simulink model "car_model"  (R2022b)
settings: Solver=VariableStepAuto  StartTime=0.0  StopTime=30  RelTol=1e-3
values from neighbouring files (symbols this model uses):
  X = Chassis_Signals.InertFrm.Cg.Disp.X.Data(:)    [Simulation_Data_Parse.m]    (also in Vehicle_Sim_Parse.m)
  Y = Chassis_Signals.InertFrm.Cg.Disp.Y.Data(:)    [Simulation_Data_Parse.m]    (also in Vehicle_Sim_Parse.m)
undefined symbols (not defined in the file or in its folder): ABS_MAX_TORQUE, ABS_MAX_TRQ_CMD, ABS_MIN_TORQUE, acc_IC, ACCELERATION_MAX, ActSuspDutyCycle, Aeq_left, Aeq_right, alpha_error, ang_acc_hystersesis, ang_IC, ang_vel_IC, area_air, axb, battery_current_IC, BATTERY_CURRENT_MAX, BATTERY_CURRENT_MIN, battery_FT_IC, battery_T_IC, BATTERY_TEMPERATURE_MAX, BATTERY_TEMPERATURE_MIN, battery_voltage_IC, BATTERY_VOLTAGE_MAX, BATTERY_VOLTAGE_MIN, Brake_Pressure_IC, ccl_IC, CENTER_STEER_ANGLE_MAX, covA, covarience_matrix_IC, covG, covM, covP, covV, cy_sweep, dB, dcl_IC, DCL_MAX, DCL_MIN, deadband_angle, dIndex, DiscIntNeverNeededParam, disk_abore, driver_t, dt_OFF, dt_ON, dTx, dx, dZ, F0z, forward_look_straight, forward_look_turn, fusion_t, fusion_t_sim, Fz_IC, Fz_sweep, g, gearbox_efficiency, gps_counter_IC, gps_ratio, gr ... (+105)
libraries: fl_lib x62, nesl_utility x16, vehdynlibtire x10, vehdynlibsuspension x8, simulink x5, autolibutils x5, sharedtransform x5, EngineCoolingComponents_lib x4, slpidlib x3, SimscapeFluids_lib x3, dspstat3 x2, shared6dof x2
(part 10 of 10)

== system car_model/Vehicle Model/Wheels and Tires/VDBS/Tires/MF Tires Vector ==
  DriveTorque : Inport
  Brake Pedal : Inport  Port=2
  r : Inport  Port=3
  Vx : Inport  Port=4
  Vy : Inport  Port=5
  Camber : Inport  Port=6
  Press : Inport  Port=7  Unit=Pa
  lambda : Inport  Port=8  Unit=1
  Gnd : Inport  Port=9
  FzSusp : Inport  Port=10
  Combined Slip Wheel 2DOF : vehdynlibtire/Combined Slip Wheel 2DOF  plySteer=on  turnslip=on  tireType=External file  BrakeType=Disc  mu_static=mu_static  mu_kinetic=mu_kinetic  disk_abore=disk_abore  Rm=Rm  num_pads=num_pads  drum_abore=0.0508  drum_a=0.123  drum_c=0.212  drum_r=0.15  drum_theta1=0  drum_theta2=126  brake_p_bpt=[1 11.4736842105263 21.9473684210526 32.4210526315789 42.8947368421053 53.3684210526316 63.8421052631579 74.3157894736842 84.7894736842105 95.2631578947368 105.736842105263 116.210526315789 126.684210526316 137.157894736842 147.631578947368 158.105263157895 168.578947368421 179.052631578947 189.526315789474 200]  brake_n_bpt=[0 52.6315789473684 105.263157894737 157.894736842105 210.526315789474 263.157894736842 315.789473684211 368.421052631579 421.052631578947 473.684210526316 526.315789473684 578.947368421053 631.578947368421 684.210526315789 736.842105263158 789.473684210526 842.105263157895 894.736842105263 947.368421052632 1000]  f_brake_t=[43.4900602404453 42.5056030554862 41.5350898940194 40.5780454442085 39.6340111501808 38.7025443887544 37.7832176914519 36.8756180088306 35.9793460143796 35.0940154454303 34.2192524787115 33.3546951383474 32.4999927342521 31.6548053290159 30.8188032315107 29.991666515561 29.1730845621415 28.362755623661 27.5603864089927 26.765691687993;498.991217495636 487.695866636631 476.560505099801 465.579679307235 454.748127933653 444.060772460445 433.51270824929 423.099196101319 412.81565427025 402.657650900201 392.620896861006 382.701238955775 372.894653477208 363.197240090814 353.605216024701 344.114910546964 334.722759712992 325.425301366216 316.219170376863 307.10109410434;954.492374750826 932.886130217776 911.585920305583 890.581313170261 869.862244717126 849.419000532136 829.242198807128 809.322774193808 789.651962526121 770.221286354971 751.0225412433 732.047782773203 713.289314220164 694.739674852612 676.391628817892 658.238154578366 640.272434863842 622.48784710877 604.877954344734 587.436496520688;1409.99353200602 1378.07639379892 1346.61133551136 1315.58294703329 1284.9763615006 1254.77722860383 1224.97168936497 1195.5463522863 1166.48827078199 1137.78492180974 1109.42418562559 1081.39432659063 1053.68397496312 1026.28210961441 999.178041611083 972.361398609768 945.822110014692 919.550392851325 893.536738312604 867.771898937035;1865.49468926121 1823.26665738007 1781.63675071715 1740.58458089631 1700.09047828407 1660.13545667552 1620.7011799228 1581.76993037878 1543.32457903786 1505.34855726451 1467.82583000789 1430.74087040806 1394.07863570608 1357.82454437621 1321.96445440427 1286.48464264117 1251.37178516554 1216.61293859388 1182.19552228048 1148.10730135338;2320.9958465164 2268.45692096121 2216.66216592293 2165.58621475934 2115.20459506754 2065.49368474721 2016.43067048064 1967.99350847127 1920.16088729373 1872.91219271928 1826.22747439018 1780.08741422549 1734.47329644903 1689.36697913801 1644.75086719747 1600.60788667257 1556.92146031639 1513.67548433643 1470.85430624835 1428.44270376973;2776.49700377159 2713.64718454235 2651.68758112871 2590.58784862237 2530.31871185102 2470.8519128189 2412.16016103848 2354.21708656376 2296.9971955496 2240.47582817405 2184.62911877248 2129.43395804292 2074.86795719199 2020.9094138998 1967.53727999066 1914.73113070398 1862.47113546724 1810.73803007899 1759.51309021622 1708.77810618608;3231.99816102678 3158.8374481235 3086.71299633449 3015.58948248539 2945.43282863449 2876.21014089059 2807.88965159632 2740.44066465625 2673.83350380547 2608.03946362882 2543.03076315477 2478.78050186034 2415.26261793494 2352.4518486616 2290.32369278385 2228.85437473538 2168.02081061809 2107.80057582154 2048.17187418409 1989.11350860242;3687.49931828197 3604.02771170464 3521.73841154027 3440.59111634842 3360.54694541796 3281.56836896228 3203.61914215416 3126.66424274874 3050.66981206134 2975.60309908359 2901.43240753707 2828.12704567777 2755.6572786779 2683.9942834234 2613.11010557704 2542.97761876678 2473.57048576894 2404.8631215641 2336.83065815196 2269.44891101877;4143.00047553716 4049.21797528579 3956.76382674606 3865.59275021144 3775.66106220143 3686.92659703397 3599.34863271199 3512.88782084123 3427.50612031721 3343.16673453836 3259.83405191936 3177.4735894952 3096.05193942085 3015.5367181852 2935.89651837023 2857.10086279818 2779.12016091979 2701.92566730665 2625.48944211983 2549.78431343512;4598.50163279235 4494.40823886693 4391.78924195184 4290.59438407447 4190.77517898491 4092.28482510566 3995.07812326983 3899.11139893372 3804.34242857308 3710.73036999313 3618.23569630166 3526.82013331263 3436.44660016381 3347.079152947 3258.68293116342 3171.22410682959 3084.66983607064 2998.98821304921 2914.1482260877 2830.11971585147;5054.00279004754 4939.59850244808 4826.81465715762 4715.59601793749 4605.88929576838 4497.64305317735 4390.80761382767 4285.3349770262 4181.17873682896 4078.2940054479 3976.63734068395 3876.16667713006 3776.84126090677 3678.62158770879 3581.46934395661 3485.34735086099 ...(+2764 chars)]  tireParamSet=C:\Users\Inver\Desktop\Round_6_Hoosier_LCO_18x6_10_on_6in_12psi_PAC02_UM4.tir  PRESMAX=1000000  PRESMIN=10000  FZMAX=10000  FZMIN=100  VXLOW=VXLOW  KPUMAX=1.5  KPUMIN=-1.5  ALPMAX=1.5  ALPMIN=-1.5  CAMMAX=0.2  CAMMIN=-0.2  LONGVL=LONGVL  FxRelFreqLwrLim=200*pi  FyRelFreqLwrLim=50*pi  MyRelFreqLwrLim=100*pi  omegao=omega_IC  br=br  UNLOADED_RADIUS=UNLOADED_RADIUS  NOMPRES=NOMPRES  FNOMIN=FNOMIN  WIDTH=WIDTH  RIM_RADIUS=RIM_RADIUS  MASS=mean(m_unsprung)  IYY=IYY  GRAVITY=-g  zo=z_tire_IC  zdoto=zdot_tires_IC  BREFF=8.25094594147963  DREFF=0.260468730454265  FREFF=0.0735298544471851  Q_RE0=1.00866439868088  Q_V1=0.000760413786224011  Q_V2=0.0463384792019201  Q_FZ1=0  Q_FZ2=15.6870832810226  Q_FZ3=0  Q_FCX=0.138643970247602  Q_FCY=0.10843499565426  Q_FCY2=-0.465763352339538  PFZ1=0.69958166705601  VERTICAL_STIFFNESS=207885.061134007  VERTICAL_DAMPING=VERTICAL_DAMPING  BOTTOM_OFFST=0.00990653336182505  BOTTOM_STIFF=1999075.87051971  LONGITUDINAL_STIFFNESS=388714.175879854  LATERAL_STIFFNESS=157087.404633332  PCFX1=0.18539229191199  PCFX2=0  PCFX3=0  PCFY1=0.163183345037677  PCFY2=0  PCFY3=0.249094918231954  Q_RA1=0.675942571700787  Q_RA2=0.73800463546164  Q_RB1=1.04487486456705  Q_RB2=-1.191763806629  PCX1=1.58523057950359  PDX1=1.0239116238178  PDX2=-0.0842405110022724  PDX3=0  PEX1=0.110312777158455  PEX2=0.313468516038146  PEX3=0  PEX4=0.0016060905760045  PKX1=21.3872544684023  PKX2=14.0006541873175  PKX3=-0.405326109653452  PHX1=0.000212599305364818  PHX2=0.00115950515263055  PVX1=1.59236164471432e-05  PVX2=0.000104321112127671  PPX1=-0.349461321276586  PPX2=0.387840040616429  PPX3=-0.0969947336569324  PPX4=0.0632271859795801  RBX1=12.7633329850276  RBX2=9.5787123658471  RBX3=0  RCX1=1.02796280922059  REX1=-0.45202516851367  REX2=-0.47304886171176  RHX1=0.000233272373115809  QSX1=-0.00788307788961443  QSX2=0.954629515459396  QSX3=0.0155855777667025  QSX4=0.125904607142414  QSX5=1.01110069703963  QSX6=20.1938577118433  QSX7=0.310818120717083  QSX8=-0.0430823751139655  QSX9=0.636494404888216  QSX10=0.142438060591663  QSX11=0.346766530036373  QSX12=0  QSX13=0  QSX14=0  PPMX1=0  PCY1=1.34299950037631  PDY1=0.878267729082195  PDY2=-0.0644597923147385  PDY3=0  PEY1=-0.809776534470972  PEY2=-0.600180598867198  PEY3=0.0991732552633487  PEY4=-6.5577974035573  PEY5=0  PKY1=-15.5714726518315  PKY2=1.73126522291751  PKY3=0.365349873517229  PKY4=1.98176755955416  PKY5=0  PKY6=-0.884005199550313  PKY7=-0.237259727611847  PHY1=-0.00183370557235628  PHY2=0.00346401302716671  PVY1=-0.00675427560163264  PVY2=0.036379218103843  PVY3=-0.163543984089166  PVY4=-0.491003349625726  PPY1=-0.62059646553185  PPY2=-0.0647824842338686  PPY3=-0.164648843290686  PPY4=0.283193909060098  PPY5=0  RBY1=10.7588809173639  RBY2=7.70420065295029  RBY3=3.40283755070691e-06  RBY4=0  RCY1=1.06691874059059  REY1=0.308244924574305  REY2=7.48775032604508e-06  RHY1=0.0118479204960415  RHY2=7.63650177161071e-06  RVY1=0.0560024425050078  RVY2=7.48487127056197e-06  RVY3=0  RVY4=98.4047026517149  RVY5=2.02759273900054  RVY6=15.7623064923347  QSY1=0.00699077564863536  QSY2=0  QSY3=0.00153535478298811  QSY4=8.55710322455322e-05  QSY5=0  QSY6=0  QSY7=0.89443879773793  QSY8=-0.403227641260894  QBZ1=11.666656027484  QBZ2=-1.30355438574485  QBZ3=0  QBZ4=0.177918305399071  QBZ5=-0.162481135068033  QBZ6=0  QBZ9=30.1445534682089  QBZ10=0  QCZ1=1.29026978207574  QDZ1=0.0886972644991399  QDZ2=-0.0058634820161856  QDZ3=0.3805597481383  QDZ4=0  QDZ6=0.00160914918118959  QDZ7=-0.00211036330862154  QDZ8=-0.13921904912557  QDZ9=0.00816585550028243  QDZ10=0  QDZ11=0  QEZ1=-2.19802254534746  QEZ2=1.01850535789165  QEZ3=0  QEZ4=0.278379679112054  QEZ5=-0.548414722765386  QHZ1=0.00148361198869669  QHZ2=0.00202017567585904  QHZ3=0.240316641332066  QHZ4=-0.210114035738085  PPZ1=-0.443927982388615  PPZ2=0  SSZ1=0.00914999585397887  SSZ2=0.0389830656052735  SSZ3=0  SSZ4=0  PDXP1=0.396718274678791  PDXP2=0  PDXP3=0  PKYP1=1.00587060633573  PDYP1=0.40483048923438  PDYP2=0  PDYP3=0  PDYP4=0  PHYP1=0.992731942067188  PHYP2=0.150352945499914  PHYP3=0  PHYP4=-3.98988682633674  PECP1=0.502379254513503  PECP2=0  QDTP1=10.0178654287947  QCRP1=0.200627747200702  QCRP2=0.0995735881599772  QBRP1=0.0997107127960717  QDRP1=1.01432910167423  QDRP2=0  aMode=2
  Terminator{7..13} (7 alike) : Terminator
  Wheels : Outport  VectorParamsAs1DForOutWhenUnconnected=off
  wires:
  lambda/1 -> Combined Slip Wheel 2DOF/10
  Combined Slip Wheel 2DOF/1 -> Wheels/1
  DriveTorque/1 -> Combined Slip Wheel 2DOF/2
  Vx/1 -> Combined Slip Wheel 2DOF/3
  Camber/1 -> Combined Slip Wheel 2DOF/5
  r/1 -> Combined Slip Wheel 2DOF/6
  Press/1 -> Combined Slip Wheel 2DOF/7
  Gnd/1 -> Combined Slip Wheel 2DOF/8
  FzSusp/1 -> Combined Slip Wheel 2DOF/9
  Combined Slip Wheel 2DOF/2 -> Terminator7/1
  Combined Slip Wheel 2DOF/3 -> Terminator8/1
  Combined Slip Wheel 2DOF/4 -> Terminator9/1
  Combined Slip Wheel 2DOF/5 -> Terminator10/1
  Combined Slip Wheel 2DOF/6 -> Terminator11/1
  Combined Slip Wheel 2DOF/7 -> Terminator12/1
  Combined Slip Wheel 2DOF/8 -> Terminator13/1
  Vy/1 -> Combined Slip Wheel 2DOF/4
  Brake Pedal/1 -> Combined Slip Wheel 2DOF/1

== system car_model/Vehicle Model/Wheels and Tires/VDBS/Veh2Tire/Wheel Angles ==
  steer : Inport
  camber : Inport  Port=2
  Constant3 : Constant  Value=ones(1,4).*0
  Reshape : Reshape  OutputDimensionality=Row vector (2-D)
  Reshape1 : Reshape  OutputDimensionality=Row vector (2-D)
  Reshape2 : Reshape  OutputDimensionality=Row vector (2-D)
  Vector Concatenate3 : Concatenate  NumInputs=3  Mode=Multidimensional array
  Vehicle : Outport  VectorParamsAs1DForOutWhenUnconnected=off
  wires:
  Constant3/1 -> Reshape2/1
  Vector Concatenate3/1 -> Vehicle/1
  Reshape/1 -> Vector Concatenate3/3
  Reshape1/1 -> Vector Concatenate3/1
  camber/1 -> Reshape1/1
  Reshape2/1 -> Vector Concatenate3/2
  steer/1 -> Reshape/1

== system car_model/Vehicle Model/Wheels and Tires/VDBS/Veh2Tire/Wheel to Body Transform ==
  VelVeh : Inport  Partition=on  PartitionDimension=2  PartitionWidth=1  PartitionOffset=0
  WheelAngles : Inport  Port=2  Partition=on  PartitionDimension=2  PartitionWidth=1  PartitionOffset=0
  Constant : Constant  Value=[pi;0;0]
  Demux1 : Demux  Outputs=3
  Divide1 : Product  Inputs=**  Multiplication=Matrix(*)
  Divide2 : Product  Inputs=**  Multiplication=Matrix(*)
  For Each : ForEach  DisableCoverage=on
  Rotation Angles to Direction Cosine Matrix : sharedtransform/Rotation Angles to Direction Cosine Matrix  rotationOrder=ZYX  aMode=2
  Rotation Angles to Direction Cosine Matrix1 : sharedtransform/Rotation Angles to Direction Cosine Matrix  rotationOrder=ZYX  aMode=2
  Selector : Selector  InputPortWidth=3  IndexOptions=Index vector (dialog)  Indices=[3 2 1]  OutputSizes=1
  Selector1 : Selector  InputPortWidth=3  IndexOptions=Index vector (dialog)  Indices=[3 2 1]  OutputSizes=1
  xdotWheel : Outport  ConcatenationDimension=1  VectorParamsAs1DForOutWhenUnconnected=off
  ydotWheel : Outport  Port=2  ConcatenationDimension=1  VectorParamsAs1DForOutWhenUnconnected=off
  zdotWheel : Outport  Port=3  ConcatenationDimension=1  VectorParamsAs1DForOutWhenUnconnected=off
  wires:
  Divide2/1 -> Demux1/1
  Demux1/1 -> xdotWheel/1
  Demux1/2 -> ydotWheel/1
  Demux1/3 -> zdotWheel/1
  Rotation Angles to Direction Cosine Matrix/1 -> Divide1/1
  VelVeh/1 -> Divide1/2
  WheelAngles/1 -> Selector/1
  Selector/1 -> Rotation Angles to Direction Cosine Matrix/1
  Selector1/1 -> Rotation Angles to Direction Cosine Matrix1/1
  Rotation Angles to Direction Cosine Matrix1/1 -> Divide2/1
  Divide1/1 -> Divide2/2
  Constant/1 -> Selector1/1

== system car_model/Vehicle Model/Wheels and Tires/VDBS/Tires/Fiala Tires/Fx ==
  In1 : Inport
  In2 : Inport  Port=2
  In3 : Inport  Port=3
  In4 : Inport  Port=4
  Bus Selector{,1..3} (4 alike) : BusSelector  OutputSignals=Fx
  Vector Concatenate : Concatenate  NumInputs=4
  Out1 : Outport  VectorParamsAs1DForOutWhenUnconnected=off
  wires:
  Bus Selector3/1 -> Vector Concatenate/4  "<Fx>"
  Bus Selector2/1 -> Vector Concatenate/3  "<Fx>"
  Bus Selector1/1 -> Vector Concatenate/2  "<Fx>"
  In4/1 -> Bus Selector3/1
  In3/1 -> Bus Selector2/1
  In2/1 -> Bus Selector1/1
  Bus Selector/1 -> Vector Concatenate/1  "<Fx>"
  In1/1 -> Bus Selector/1
  Vector Concatenate/1 -> Out1/1

== system car_model/Vehicle Model/Wheels and Tires/VDBS/Tires/Fiala Tires/Fy ==
  In1 : Inport
  In2 : Inport  Port=2
  In3 : Inport  Port=3
  In4 : Inport  Port=4
  Bus Selector{,1..3} (4 alike) : BusSelector  OutputSignals=Fy
  Vector Concatenate : Concatenate  NumInputs=4
  Out1 : Outport  VectorParamsAs1DForOutWhenUnconnected=off
  wires:
  Vector Concatenate/1 -> Out1/1
  In1/1 -> Bus Selector/1
  Bus Selector/1 -> Vector Concatenate/1  "<Fy>"
  In2/1 -> Bus Selector1/1
  In3/1 -> Bus Selector2/1
  In4/1 -> Bus Selector3/1
  Bus Selector1/1 -> Vector Concatenate/2  "<Fy>"
  Bus Selector2/1 -> Vector Concatenate/3  "<Fy>"
  Bus Selector3/1 -> Vector Concatenate/4  "<Fy>"

== system car_model/Vehicle Model/Wheels and Tires/VDBS/Tires/Fiala Tires/Fz ==
  In1 : Inport
  In2 : Inport  Port=2
  In3 : Inport  Port=3
  In4 : Inport  Port=4
  Bus Selector{,1..3} (4 alike) : BusSelector  OutputSignals=Fz
  Vector Concatenate : Concatenate  NumInputs=4
  Out1 : Outport  VectorParamsAs1DForOutWhenUnconnected=off
  wires:
  Vector Concatenate/1 -> Out1/1
  In1/1 -> Bus Selector/1
  Bus Selector/1 -> Vector Concatenate/1  "<Fz>"
  In2/1 -> Bus Selector1/1
  In3/1 -> Bus Selector2/1
  In4/1 -> Bus Selector3/1
  Bus Selector1/1 -> Vector Concatenate/2  "<Fz>"
  Bus Selector2/1 -> Vector Concatenate/3  "<Fz>"
  Bus Selector3/1 -> Vector Concatenate/4  "<Fz>"

== system car_model/Vehicle Model/Wheels and Tires/VDBS/Tires/Fiala Tires/Mx ==
  In1 : Inport
  In2 : Inport  Port=2
  In3 : Inport  Port=3
  In4 : Inport  Port=4
  Bus Selector{,1..3} (4 alike) : BusSelector  OutputSignals=Mx
  Vector Concatenate : Concatenate  NumInputs=4
  Out1 : Outport  VectorParamsAs1DForOutWhenUnconnected=off
  wires:
  Vector Concatenate/1 -> Out1/1
  In1/1 -> Bus Selector/1
  Bus Selector/1 -> Vector Concatenate/1  "<Mx>"
  In2/1 -> Bus Selector1/1
  In3/1 -> Bus Selector2/1
  In4/1 -> Bus Selector3/1
  Bus Selector1/1 -> Vector Concatenate/2  "<Mx>"
  Bus Selector2/1 -> Vector Concatenate/3  "<Mx>"
  Bus Selector3/1 -> Vector Concatenate/4  "<Mx>"

== system car_model/Vehicle Model/Wheels and Tires/VDBS/Tires/Fiala Tires/My ==
  In1 : Inport
  In2 : Inport  Port=2
  In3 : Inport  Port=3
  In4 : Inport  Port=4
  Bus Selector{,1..3} (4 alike) : BusSelector  OutputSignals=My
  Vector Concatenate : Concatenate  NumInputs=4
  Out1 : Outport  VectorParamsAs1DForOutWhenUnconnected=off
  wires:
  Bus Selector3/1 -> Vector Concatenate/4  "<My>"
  Bus Selector2/1 -> Vector Concatenate/3  "<My>"
  Bus Selector1/1 -> Vector Concatenate/2  "<My>"
  In4/1 -> Bus Selector3/1
  In3/1 -> Bus Selector2/1
  In2/1 -> Bus Selector1/1
  Bus Selector/1 -> Vector Concatenate/1  "<My>"
  In1/1 -> Bus Selector/1
  Vector Concatenate/1 -> Out1/1

== system car_model/Vehicle Model/Wheels and Tires/VDBS/Tires/Fiala Tires/Mz ==
  In1 : Inport
  In2 : Inport  Port=2
  In3 : Inport  Port=3
  In4 : Inport  Port=4
  Bus Selector{,1..3} (4 alike) : BusSelector  OutputSignals=Mz
  Vector Concatenate : Concatenate  NumInputs=4
  Out1 : Outport  VectorParamsAs1DForOutWhenUnconnected=off
  wires:
  Bus Selector3/1 -> Vector Concatenate/4  "<Mz>"
  Bus Selector2/1 -> Vector Concatenate/3  "<Mz>"
  Bus Selector1/1 -> Vector Concatenate/2  "<Mz>"
  In4/1 -> Bus Selector3/1
  In3/1 -> Bus Selector2/1
  In2/1 -> Bus Selector1/1
  Bus Selector/1 -> Vector Concatenate/1  "<Mz>"
  In1/1 -> Bus Selector/1
  Vector Concatenate/1 -> Out1/1

== system car_model/Vehicle Model/Wheels and Tires/VDBS/Tires/Fiala Tires/Re ==
  In1 : Inport
  In2 : Inport  Port=2
  In3 : Inport  Port=3
  In4 : Inport  Port=4
  Bus Selector{,1..3} (4 alike) : BusSelector  OutputSignals=Re
  Vector Concatenate : Concatenate  NumInputs=4
  Out1 : Outport  VectorParamsAs1DForOutWhenUnconnected=off
  wires:
  Vector Concatenate/1 -> Out1/1
  In1/1 -> Bus Selector/1
  Bus Selector/1 -> Vector Concatenate/1  "<Re>"
  In2/1 -> Bus Selector1/1
  In3/1 -> Bus Selector2/1
  In4/1 -> Bus Selector3/1
  Bus Selector1/1 -> Vector Concatenate/2  "<Re>"
  Bus Selector2/1 -> Vector Concatenate/3  "<Re>"
  Bus Selector3/1 -> Vector Concatenate/4  "<Re>"

== system car_model/Vehicle Model/Wheels and Tires/VDBS/Tires/Fiala Tires/alpha ==
  In1 : Inport
  In2 : Inport  Port=2
  In3 : Inport  Port=3
  In4 : Inport  Port=4
  Bus Selector{,1..3} (4 alike) : BusSelector  OutputSignals=Alpha
  Vector Concatenate : Concatenate  NumInputs=4
  Out1 : Outport  VectorParamsAs1DForOutWhenUnconnected=off
  wires:
  Vector Concatenate/1 -> Out1/1
  In1/1 -> Bus Selector/1
  Bus Selector/1 -> Vector Concatenate/1  "<Alpha>"
  In2/1 -> Bus Selector1/1
  In3/1 -> Bus Selector2/1
  In4/1 -> Bus Selector3/1
  Bus Selector1/1 -> Vector Concatenate/2  "<Alpha>"
  Bus Selector2/1 -> Vector Concatenate/3  "<Alpha>"
  Bus Selector3/1 -> Vector Concatenate/4  "<Alpha>"

== system car_model/Vehicle Model/Wheels and Tires/VDBS/Tires/Fiala Tires/kappa ==
  In1 : Inport
  In2 : Inport  Port=2
  In3 : Inport  Port=3
  In4 : Inport  Port=4
  Bus Selector{,1..3} (4 alike) : BusSelector  OutputSignals=Kappa
  Vector Concatenate : Concatenate  NumInputs=4
  Out1 : Outport  VectorParamsAs1DForOutWhenUnconnected=off
  wires:
  Bus Selector3/1 -> Vector Concatenate/4  "<Kappa>"
  Bus Selector2/1 -> Vector Concatenate/3  "<Kappa>"
  Bus Selector1/1 -> Vector Concatenate/2  "<Kappa>"
  In4/1 -> Bus Selector3/1
  In3/1 -> Bus Selector2/1
  In2/1 -> Bus Selector1/1
  Bus Selector/1 -> Vector Concatenate/1  "<Kappa>"
  In1/1 -> Bus Selector/1
  Vector Concatenate/1 -> Out1/1

== system car_model/Vehicle Model/Wheels and Tires/VDBS/Tires/Fiala Tires/omega ==
  In1 : Inport
  In2 : Inport  Port=2
  In3 : Inport  Port=3
  In4 : Inport  Port=4
  Bus Selector{,1..3} (4 alike) : BusSelector  OutputSignals=Omega
  Vector Concatenate : Concatenate  NumInputs=4
  Out1 : Outport  VectorParamsAs1DForOutWhenUnconnected=off
  wires:
  In1/1 -> Bus Selector/1
  Bus Selector/1 -> Vector Concatenate/1  "<Omega>"
  In2/1 -> Bus Selector1/1
  In3/1 -> Bus Selector2/1
  In4/1 -> Bus Selector3/1
  Bus Selector1/1 -> Vector Concatenate/2  "<Omega>"
  Bus Selector2/1 -> Vector Concatenate/3  "<Omega>"
  Bus Selector3/1 -> Vector Concatenate/4  "<Omega>"
  Vector Concatenate/1 -> Out1/1

== system car_model/Vehicle Model/Wheels and Tires/VDBS/Tires/Fiala Tires/z ==
  In1 : Inport
  In2 : Inport  Port=2
  In3 : Inport  Port=3
  In4 : Inport  Port=4
  Bus Selector{,1..3} (4 alike) : BusSelector  OutputSignals=z
  Vector Concatenate : Concatenate  NumInputs=4
  Out1 : Outport  VectorParamsAs1DForOutWhenUnconnected=off
  wires:
  Bus Selector3/1 -> Vector Concatenate/4  "<z>"
  Bus Selector2/1 -> Vector Concatenate/3  "<z>"
  Bus Selector1/1 -> Vector Concatenate/2  "<z>"
  In4/1 -> Bus Selector3/1
  In3/1 -> Bus Selector2/1
  In2/1 -> Bus Selector1/1
  Bus Selector/1 -> Vector Concatenate/1  "<z>"
  In1/1 -> Bus Selector/1
  Vector Concatenate/1 -> Out1/1

== system car_model/Vehicle Model/Wheels and Tires/VDBS/Tires/Fiala Tires/zdot ==
  In1 : Inport
  In2 : Inport  Port=2
  In3 : Inport  Port=3
  In4 : Inport  Port=4
  Bus Selector{,1..3} (4 alike) : BusSelector  OutputSignals=zdot
  Vector Concatenate : Concatenate  NumInputs=4
  Out1 : Outport  VectorParamsAs1DForOutWhenUnconnected=off
  wires:
  Vector Concatenate/1 -> Out1/1
  In1/1 -> Bus Selector/1
  Bus Selector/1 -> Vector Concatenate/1  "<zdot>"
  In2/1 -> Bus Selector1/1
  In3/1 -> Bus Selector2/1
  In4/1 -> Bus Selector3/1
  Bus Selector1/1 -> Vector Concatenate/2  "<zdot>"
  Bus Selector2/1 -> Vector Concatenate/3  "<zdot>"
  Bus Selector3/1 -> Vector Concatenate/4  "<zdot>"

== system car_model/Vehicle Model/Wheels and Tires/VDBS/Tires/MF Tires/Fx ==
  In1 : Inport
  In2 : Inport  Port=2
  In3 : Inport  Port=3
  In4 : Inport  Port=4
  Bus Selector{,1..3} (4 alike) : BusSelector  OutputSignals=Fx
  Vector Concatenate : Concatenate  NumInputs=4
  Out1 : Outport  VectorParamsAs1DForOutWhenUnconnected=off
  wires:
  Bus Selector3/1 -> Vector Concatenate/4  "<Fx>"
  Bus Selector2/1 -> Vector Concatenate/3  "<Fx>"
  Bus Selector1/1 -> Vector Concatenate/2  "<Fx>"
  In4/1 -> Bus Selector3/1
  In3/1 -> Bus Selector2/1
  In2/1 -> Bus Selector1/1
  Bus Selector/1 -> Vector Concatenate/1  "<Fx>"
  In1/1 -> Bus Selector/1
  Vector Concatenate/1 -> Out1/1

== system car_model/Vehicle Model/Wheels and Tires/VDBS/Tires/MF Tires/Fy ==
  In1 : Inport
  In2 : Inport  Port=2
  In3 : Inport  Port=3
  In4 : Inport  Port=4
  Bus Selector{,1..3} (4 alike) : BusSelector  OutputSignals=Fy
  Vector Concatenate : Concatenate  NumInputs=4
  Out1 : Outport  VectorParamsAs1DForOutWhenUnconnected=off
  wires:
  Vector Concatenate/1 -> Out1/1
  In1/1 -> Bus Selector/1
  Bus Selector/1 -> Vector Concatenate/1  "<Fy>"
  In2/1 -> Bus Selector1/1
  In3/1 -> Bus Selector2/1
  In4/1 -> Bus Selector3/1
  Bus Selector1/1 -> Vector Concatenate/2  "<Fy>"
  Bus Selector2/1 -> Vector Concatenate/3  "<Fy>"
  Bus Selector3/1 -> Vector Concatenate/4  "<Fy>"

== system car_model/Vehicle Model/Wheels and Tires/VDBS/Tires/MF Tires/Fz ==
  In1 : Inport
  In2 : Inport  Port=2
  In3 : Inport  Port=3
  In4 : Inport  Port=4
  Bus Selector{,1..3} (4 alike) : BusSelector  OutputSignals=Fz
  Vector Concatenate : Concatenate  NumInputs=4
  Out1 : Outport  VectorParamsAs1DForOutWhenUnconnected=off
  wires:
  Vector Concatenate/1 -> Out1/1
  In1/1 -> Bus Selector/1
  Bus Selector/1 -> Vector Concatenate/1  "<Fz>"
  In2/1 -> Bus Selector1/1
  In3/1 -> Bus Selector2/1
  In4/1 -> Bus Selector3/1
  Bus Selector1/1 -> Vector Concatenate/2  "<Fz>"
  Bus Selector2/1 -> Vector Concatenate/3  "<Fz>"
  Bus Selector3/1 -> Vector Concatenate/4  "<Fz>"

== system car_model/Vehicle Model/Wheels and Tires/VDBS/Tires/MF Tires/Mx ==
  In1 : Inport
  In2 : Inport  Port=2
  In3 : Inport  Port=3
  In4 : Inport  Port=4
  Bus Selector{,1..3} (4 alike) : BusSelector  OutputSignals=Mx
  Vector Concatenate : Concatenate  NumInputs=4
  Out1 : Outport  VectorParamsAs1DForOutWhenUnconnected=off
  wires:
  Vector Concatenate/1 -> Out1/1
  In1/1 -> Bus Selector/1
  Bus Selector/1 -> Vector Concatenate/1  "<Mx>"
  In2/1 -> Bus Selector1/1
  In3/1 -> Bus Selector2/1
  In4/1 -> Bus Selector3/1
  Bus Selector1/1 -> Vector Concatenate/2  "<Mx>"
  Bus Selector2/1 -> Vector Concatenate/3  "<Mx>"
  Bus Selector3/1 -> Vector Concatenate/4  "<Mx>"

== system car_model/Vehicle Model/Wheels and Tires/VDBS/Tires/MF Tires/My ==
  In1 : Inport
  In2 : Inport  Port=2
  In3 : Inport  Port=3
  In4 : Inport  Port=4
  Bus Selector{,1..3} (4 alike) : BusSelector  OutputSignals=My
  Vector Concatenate : Concatenate  NumInputs=4
  Out1 : Outport  VectorParamsAs1DForOutWhenUnconnected=off
  wires:
  Bus Selector3/1 -> Vector Concatenate/4  "<My>"
  Bus Selector2/1 -> Vector Concatenate/3  "<My>"
  Bus Selector1/1 -> Vector Concatenate/2  "<My>"
  In4/1 -> Bus Selector3/1
  In3/1 -> Bus Selector2/1
  In2/1 -> Bus Selector1/1
  Bus Selector/1 -> Vector Concatenate/1  "<My>"
  In1/1 -> Bus Selector/1
  Vector Concatenate/1 -> Out1/1

== system car_model/Vehicle Model/Wheels and Tires/VDBS/Tires/MF Tires/Mz ==
  In1 : Inport
  In2 : Inport  Port=2
  In3 : Inport  Port=3
  In4 : Inport  Port=4
  Bus Selector{,1..3} (4 alike) : BusSelector  OutputSignals=Mz
  Vector Concatenate : Concatenate  NumInputs=4
  Out1 : Outport  VectorParamsAs1DForOutWhenUnconnected=off
  wires:
  Bus Selector3/1 -> Vector Concatenate/4  "<Mz>"
  Bus Selector2/1 -> Vector Concatenate/3  "<Mz>"
  Bus Selector1/1 -> Vector Concatenate/2  "<Mz>"
  In4/1 -> Bus Selector3/1
  In3/1 -> Bus Selector2/1
  In2/1 -> Bus Selector1/1
  Bus Selector/1 -> Vector Concatenate/1  "<Mz>"
  In1/1 -> Bus Selector/1
  Vector Concatenate/1 -> Out1/1

== system car_model/Vehicle Model/Wheels and Tires/VDBS/Tires/MF Tires/Re ==
  In1 : Inport
  In2 : Inport  Port=2
  In3 : Inport  Port=3
  In4 : Inport  Port=4
  Bus Selector{,1..3} (4 alike) : BusSelector  OutputSignals=Re
  Vector Concatenate : Concatenate  NumInputs=4
  Out1 : Outport  VectorParamsAs1DForOutWhenUnconnected=off
  wires:
  Vector Concatenate/1 -> Out1/1
  In1/1 -> Bus Selector/1
  Bus Selector/1 -> Vector Concatenate/1  "<Re>"
  In2/1 -> Bus Selector1/1
  In3/1 -> Bus Selector2/1
  In4/1 -> Bus Selector3/1
  Bus Selector1/1 -> Vector Concatenate/2  "<Re>"
  Bus Selector2/1 -> Vector Concatenate/3  "<Re>"
  Bus Selector3/1 -> Vector Concatenate/4  "<Re>"

== system car_model/Vehicle Model/Wheels and Tires/VDBS/Tires/MF Tires/alpha ==
  In1 : Inport
  In2 : Inport  Port=2
  In3 : Inport  Port=3
  In4 : Inport  Port=4
  Bus Selector{,1..3} (4 alike) : BusSelector  OutputSignals=Alpha
  Vector Concatenate : Concatenate  NumInputs=4
  Out1 : Outport  VectorParamsAs1DForOutWhenUnconnected=off
  wires:
  Vector Concatenate/1 -> Out1/1
  In1/1 -> Bus Selector/1
  Bus Selector/1 -> Vector Concatenate/1  "<Alpha>"
  In2/1 -> Bus Selector1/1
  In3/1 -> Bus Selector2/1
  In4/1 -> Bus Selector3/1
  Bus Selector1/1 -> Vector Concatenate/2  "<Alpha>"
  Bus Selector2/1 -> Vector Concatenate/3  "<Alpha>"
  Bus Selector3/1 -> Vector Concatenate/4  "<Alpha>"

== system car_model/Vehicle Model/Wheels and Tires/VDBS/Tires/MF Tires/kappa ==
  In1 : Inport
  In2 : Inport  Port=2
  In3 : Inport  Port=3
  In4 : Inport  Port=4
  Bus Selector{,1..3} (4 alike) : BusSelector  OutputSignals=Kappa
  Vector Concatenate : Concatenate  NumInputs=4
  Out1 : Outport  VectorParamsAs1DForOutWhenUnconnected=off
  wires:
  Bus Selector3/1 -> Vector Concatenate/4  "<Kappa>"
  Bus Selector2/1 -> Vector Concatenate/3  "<Kappa>"
  Bus Selector1/1 -> Vector Concatenate/2  "<Kappa>"
  In4/1 -> Bus Selector3/1
  In3/1 -> Bus Selector2/1
  In2/1 -> Bus Selector1/1
  Bus Selector/1 -> Vector Concatenate/1  "<Kappa>"
  In1/1 -> Bus Selector/1
  Vector Concatenate/1 -> Out1/1

== system car_model/Vehicle Model/Wheels and Tires/VDBS/Tires/MF Tires/omega ==
  In1 : Inport
  In2 : Inport  Port=2
  In3 : Inport  Port=3
  In4 : Inport  Port=4
  Bus Selector{,1..3} (4 alike) : BusSelector  OutputSignals=Omega
  Vector Concatenate : Concatenate  NumInputs=4
  Out1 : Outport  VectorParamsAs1DForOutWhenUnconnected=off
  wires:
  In1/1 -> Bus Selector/1
  Bus Selector/1 -> Vector Concatenate/1  "<Omega>"
  In2/1 -> Bus Selector1/1
  In3/1 -> Bus Selector2/1
  In4/1 -> Bus Selector3/1
  Bus Selector1/1 -> Vector Concatenate/2  "<Omega>"
  Bus Selector2/1 -> Vector Concatenate/3  "<Omega>"
  Bus Selector3/1 -> Vector Concatenate/4  "<Omega>"
  Vector Concatenate/1 -> Out1/1

== system car_model/Vehicle Model/Wheels and Tires/VDBS/Tires/MF Tires/z ==
  In1 : Inport
  In2 : Inport  Port=2
  In3 : Inport  Port=3
  In4 : Inport  Port=4
  Bus Selector{,1..3} (4 alike) : BusSelector  OutputSignals=z
  Vector Concatenate : Concatenate  NumInputs=4
  Out1 : Outport  VectorParamsAs1DForOutWhenUnconnected=off
  wires:
  Bus Selector3/1 -> Vector Concatenate/4  "<z>"
  Bus Selector2/1 -> Vector Concatenate/3  "<z>"
  Bus Selector1/1 -> Vector Concatenate/2  "<z>"
  In4/1 -> Bus Selector3/1
  In3/1 -> Bus Selector2/1
  In2/1 -> Bus Selector1/1
  Bus Selector/1 -> Vector Concatenate/1  "<z>"
  In1/1 -> Bus Selector/1
  Vector Concatenate/1 -> Out1/1

== system car_model/Vehicle Model/Wheels and Tires/VDBS/Tires/MF Tires/zdot ==
  In1 : Inport
  In2 : Inport  Port=2
  In3 : Inport  Port=3
  In4 : Inport  Port=4
  Bus Selector{,1..3} (4 alike) : BusSelector  OutputSignals=zdot
  Vector Concatenate : Concatenate  NumInputs=4
  Out1 : Outport  VectorParamsAs1DForOutWhenUnconnected=off
  wires:
  Vector Concatenate/1 -> Out1/1
  In1/1 -> Bus Selector/1
  Bus Selector/1 -> Vector Concatenate/1  "<zdot>"
  In2/1 -> Bus Selector1/1
  In3/1 -> Bus Selector2/1
  In4/1 -> Bus Selector3/1
  Bus Selector1/1 -> Vector Concatenate/2  "<zdot>"
  Bus Selector2/1 -> Vector Concatenate/3  "<zdot>"
  Bus Selector3/1 -> Vector Concatenate/4  "<zdot>"

== matlab function car_model/Vehicle Model/Vehicle/6DOF/Suspension to Chasiss Transforms/Estimated Unsprung Mass Orientation ==
  data: angles output size=3; angleIn input size=3; GeomXYZ output size=3; GemoXYZIn input size=3; Ground input size=4; trackW parameter; wheelB parameter
function [angles,GeomXYZ]= three26(angleIn, GemoXYZIn, Ground,trackW, wheelB)%#codegen
coder.allowpcode('plain')
% Copyright 2018 The MathWorks, Inc.
[angles,GeomXYZ]= vdynthree2six(angleIn, GemoXYZIn, Ground,trackW, wheelB);

== matlab function car_model/Driver & Environment/Reference Generator/Reference Geneator ==
  data: sign_distance output; index_all output; min_d output; index_small input size=1; index_all input size=1; psi input; deg2rad parameter; Vg input; yaw input; pos input; omega input; index_small output size=1; d_error output; psi_error output; v_error output; v_cog output; r_ref output; r_error output; x_ref output; y_ref output; yaw_ref output; omega output; p_error output; Vnow output; ahead output; ahead input; selected_track parameter; dIndex parameter; dx parameter; forward_look_straight parameter; forward_look_turn parameter; q_thresh parameter; indicies parameter; selected_maxvm parameter; axb parameter; di_now output; di_prev input
function [sign_distance,index_all, min_d,index_small, d_error, psi_error, v_error, v_cog, r_ref, r_error, x_ref, y_ref, yaw_ref, omega, p_error,Vnow, ahead, di_now] = ref_gen(index_small, index_all, psi, deg2rad, Vg, yaw, pos, omega, ahead, selected_track, dIndex, dx, forward_look_straight, forward_look_turn, q_thresh, indicies, selected_maxvm, axb, di_prev)
%% Extract Data
Y_all = selected_track(index_all:index_all+dIndex,2);
X_all = selected_track(index_all:index_all+dIndex,3);

Vmax_now = selected_maxvm(index_small,3);
num_elem = length(selected_maxvm(:,1));

if num_elem > index_small
    Vmax_next = selected_maxvm(index_small+1,3);
    d_next = selected_maxvm(index_small+1,1);
else
    Vmax_next = Vmax_now;
    d_next = 100;
end

%% Determine Reference Point
d_error_all = sqrt((Y_all - pos.Y).^2 + (X_all - pos.X).^2);
[min_d, min_index] = min(d_error_all);
index_all = index_all + min_index - 1;

%% Aquire Reference Values
y_ref = selected_track(index_all, 2);
x_ref = selected_track(index_all, 3);
y_ref_next = selected_track(index_all+5, 2);
x_ref_next = selected_track(index_all+5, 3);
r_ref = selected_track(index_all, 4);
r_straight = selected_track(index_all+forward_look_straight, 4);
r_turn = selected_track(index_all+forward_look_turn, 4);
turn_ref = selected_track(index_all, 5);
straight_next = selected_track(index_all+forward_look_straight, 5);
turn_next = selected_track(index_all+forward_look_turn, 5);
psi_ref = selected_track(index_all, 8);
di_now = selected_track(index_all, 9);

%% Velocity Error
v_cog = sqrt((Vg.xdot^2) + (Vg.ydot^2));

if ahead
    di = (di_now*dx) + d_next;
else
    di = di_now*dx;
end

det = v_cog^2 + (2*axb*di);

if det < 0
    Vnext = 0;
else
    Vnext = sqrt(det);
end

% straight driving simulation
% d_now = pos.X;
% d_later = selected_maxvm(index_small,4);
% dS = d_now - d_later;
% det = v_cog^2 - (2*axb*dS);
% 
% if det > 0
%     Vnext = sqrt(det);
% else
%     Vnext = 0;
% end

increment = 0;

if (abs(Vmax_next - Vnext) < 0.25) && (Vmax_now > Vmax_next) && (~ahead)% && (ahead)
    Vnow = Vmax_next;
    index_small = index_small + 1;
    ahead = 1;
    increment = 1;
elseif ((di_now - di_prev) > 0) && ~ahead
    Vnow = Vmax_next;
    index_small = index_small + 1;
else
    Vnow = Vmax_now;
end

if ((di_now - di_prev) > 0) && ~increment
    ahead = 0;
end

% if (Vnext + 0.5 < Vnow) && (selected_maxvm(index_small,1) ~= 40)
%     Vnow = 50;
% end

v_error = Vnow - v_cog;

%% Turning Radius Error
if (turn_ref ~= straight_next) || (r_ref ~= r_straight)
    turn_ref = straight_next;
    r_ref = r_straight;
elseif (turn_ref ~= turn_next) && (turn_next ~= 0) && (turn_ref ~= 0)
    turn_ref = turn_next;
    r_ref = r_turn;
end

r_IC = abs(v_cog / yaw);
r_error = turn_ref *  ((1 / r_ref) - (1 / r_IC));

if r_ref == inf
    yaw_ref = 0;
else
    yaw_ref = turn_ref * v_cog / r_ref;
end

%% Angle Error
sign_steer = 1;

if (abs(psi - psi_ref) > pi) && (sign(psi) ~= sign(psi_ref))
    if psi < 0
        sign_steer = -1;
    end
elseif (psi > psi_ref)
    sign_steer = -1;   
end

if abs(psi_ref - psi) < pi
    psi_error = sign_steer * abs(psi_ref - psi) / deg2rad;
else
    psi_error = sign_steer * ((pi - abs(psi_ref)) + (pi - abs(psi))) / deg2rad;
end

%% Distance Error
% Determine Vehicle Quadrant
if (pos.Y - y_ref) > q_thresh
   if (pos.X - x_ref) > q_thresh
       Qc = 5;
   elseif (pos.X - x_ref) < -q_thresh
       Qc = 11;
   else
       Qc = 4;
   end
elseif (pos.Y - y_ref) < -q_thresh
   if (pos.X - x_ref) > q_thresh
       Qc = 7;
   elseif (pos.X - x_ref) < -q_thresh
       Qc = 9;
   else
       Qc = 8;
   end
else
   if (pos.X - x_ref) > q_thresh
       Qc = 6;
   elseif (pos.X - x_ref) < -q_thresh
       Qc = 10;
   else
       Qc = 0;
   end
end

% Determine Next Reference Point Quadrant
if y_ref_next > y_ref
   if x_ref_next > x_ref
       Qn = 5;
   elseif x_ref_next < x_ref
       Qn = 11;
   else
       Qn = 4;
   end
elseif y_ref_next < y_ref
   if x_ref_next > x_ref
       Qn = 7;
   elseif x_ref_next < x_ref
       Qn = 9;
   else
       Qn = 8;
   end
else
   if x_ref_next > x_ref
       Qn = 6;
   elseif x_ref_next < x_ref
       Qn = 10;
   else
       Qn = 0;
   end
end

% Determine Sign for Distance Error
if Qc == 0
   sign_distance = 0;
elseif (abs(x_ref_next - x_ref) == abs(pos.X - x_ref)) && (abs(y_ref_next - y_ref) == abs(pos.Y - y_ref))
   sign_distance = 0;
elseif ((Qc ~= Qn) && (indicies(Qc+4) ~= Qn))
    if (indicies(Qc+1) == indicies(Qn)) || (indicies(Qc+2) == indicies(Qn)) || (indicies(Qc+3) == indicies(Qn))
        sign_distance = -1;
    else
        sign_distance = 1;
    end
else
    if indicies(Qc) == 1 || indicies(Qc) == 3
        y_axis = y_ref;
    elseif indicies(Qc) == 4
        y_axis = y_ref + 1;
    else
        y_axis = y_ref - 1;
    end
    
    if indicies(Qc) == 2 || indicies(Qc) == 4
        x_axis = x_ref;
    elseif indicies(Qc) == 1
        x_axis = x_ref + 1;
    else
        x_axis = x_ref - 1;
    end
    
    axis_coordiantes = [y_axis, x_axis];
    ref_coordiantes = [y_ref, x_ref];
    next_ref_coordinates = [y_ref_next, x_ref_next];
    vehicle_coordinates = [pos.Y, pos.X];
    
    ref_vec = axis_coordiantes - ref_coordiantes;
    veh_vec = vehicle_coordinates - ref_coordiantes;
    next_ref = next_ref_coordinates - ref_coordiantes;
    
    theta_veh_ref = acos(dot(ref_vec, veh_vec) / (norm(ref_vec)*norm(veh_vec)));
    theta_next_ref = acos(dot(ref_vec, next_ref) / (norm(ref_vec)*norm(next_ref)));
    
    if theta_veh_ref < theta_next_ref
        sign_distance = 1;
    else
        sign_distance = -1;
    end
end

d_error = sign_distance * min_d;

%% Combined Purtubation Error
if (sign_distance~=sign(psi_error)) && (d_error~=0)
    p_error = d_error;
else
    p_error = psi_error;
end

end

== matlab function car_model/Driver & Environment/Sweep Generator/Sweep Generator ==
  data: index input; index output; vel input; ON input; vel_err output; ref_steer output; ON output; selected_sweep parameter; dt_ON parameter; dt_OFF parameter; counter output; counter input; tvs_t_sim parameter
function [index, vel_err,ref_steer, ON, counter] = fcn(index, vel, ON, selected_sweep, dt_ON, dt_OFF, counter, tvs_t_sim)

% Update Control Output
ref_vel = selected_sweep(index, 1);
ref_steer = selected_sweep(index, 2);
vel_err = ref_vel - norm([vel.xdot vel.ydot]);
counter = counter + 1;

% Update Scenario
if ((counter*tvs_t_sim) == dt_ON && ON) || ((counter*tvs_t_sim) == dt_OFF && ~ON)
    index = index + 1;
    counter = 0;

    if (selected_sweep(index, 2) == 0 && index > 1)
        ON = double(~ON);
    end

end

== matlab function car_model/Vehicle Model/Vehicle/6DOF/Suspension to Chasiss Transforms/MATLAB Function ==
  data: u input; y output; aero_coeff parameter
function y = fcn(u, aero_coeff)

Fz = aero_coeff*u^2;


y = [0 0 Fz];

== matlab function car_model/Vehicle Model/Electronics/Navigation Sensors/VNED to SNED ==
  data: accel_SNED output; gyro_SNED output; accel_VNED input size=[3 1]; gyro_VNED input size=[3 1]; mag_VNED input size=[3 1]; mag_SNED output; phi parameter
function [accel_SNED, gyro_SNED, mag_SNED] = VNED2SNED(accel_VNED, gyro_VNED, mag_VNED, phi)
%% Define Rotation
IMUNED2VNED = rotmat(quaternion([0 (phi - 180) 0],"eulerd","XYZ","frame"),"frame");
MAGNED2VNED = rotmat(quaternion([180 (180 - phi) 0],"eulerd","XYZ","frame"),"frame");

%% Coordinate Transformation
accel_SNED = IMUNED2VNED\accel_VNED;
gyro_SNED = IMUNED2VNED\gyro_VNED;
mag_SNED = MAGNED2VNED\mag_VNED;

end

== matlab function car_model/Vehicle Model/Electronics/Navigation Sensors/integrate angvel ==
  data: Orientation_e input; Orientation_c output; Orientation_e output
function [Orientation_c, Orientation_e]  = fcn(Orientation_e)

Orientation_q = quaternion(Orientation_e', 'euler', 'XYZ', 'frame');

Orientation_c = compact(Orientation_q);

end

== matlab function car_model/Control Systems/Sensor Fusion/fusion ==
  data: count input; count output; rot_map output; velocity input size=[1,3]; state_out output; position input size=[1,3]; acceleration input size=[1,3]; angularVelocity input size=[1,3]; magField input size=[1,3]; state_in input; cov_in input; covG parameter; covA parameter; covM parameter; covP parameter; covV parameter; fusion_t parameter; location_lla_IC parameter; cov_out output; noise_state parameter; gps_ratio parameter
function [count, rot_map, state_out, cov_out] = fusion(count, velocity, position ,acceleration,angularVelocity, magField, state_in, cov_in, covG, covA, covM, covP, covV, fusion_t, location_lla_IC, noise_state, gps_ratio) 
%% Create Filter
filter = insfilterAsync();
filter.ReferenceLocation = location_lla_IC;
filter.State = state_in;
filter.StateCovariance = cov_in;

filter.QuaternionNoise = noise_state(1:4);
filter.AngularVelocityNoise = noise_state(5:7);
filter.PositionNoise = noise_state(8:10);
filter.VelocityNoise = noise_state(11:13);
filter.AccelerationNoise = noise_state(14:16);
filter.GyroscopeBiasNoise = noise_state(17:19);
filter.AccelerometerBiasNoise = noise_state(20:22);
filter.GeomagneticVectorNoise = noise_state(23:25);
filter.MagnetometerBiasNoise = noise_state(26:28);

%% Sensor Fusion
predict(filter, fusion_t);

fuseaccel(filter,acceleration,covA);
fusegyro(filter,angularVelocity,covG);
fusemag(filter, magField,covM);

if ~count
    fusegps(filter,position,covP,velocity,covV);
end

count = mod(count + 1, gps_ratio);

[~,rot_map,~] = pose(filter, 'rotmat');

%% Save Fusion State & State Covariance
state_out = filter.State;
cov_out = filter.StateCovariance;

end

== matlab function car_model/Control Systems/Sensor Fusion/NED2VNED ==
  data: rot_map input; state input; ang output; angvel output; pos output; vel output; accel output; mag output; accel_bias output; gyro_bias output; mag_bias output
function [ang,angvel,pos,vel,accel,mag,accel_bias,gyro_bias,mag_bias] = NED2VNED(rot_map, state)
%% Vehicle POSE
ang = state(1:4);                    % quaternion (VNED2SNED)
angvel = state(5:7);                 % chassis angular velocity (rad/s)(VNED)
pos = state(8:10);                   % chassis position (m)(NED)
vel = rot_map*state(11:13);          % chassis velocity (m/s)(VNED)
accel = rot_map*state(14:16);        % chassis acceleration (m/s^2)(VNED)
mag = state(23:25);                  % magnetic field (uT)(NED)

%% Sensor Parameters
accel_bias = rot_map*state(17:19);   % accelerometer bias (m/s^2)(VNED)
gyro_bias = rot_map*state(20:22);    % gyroscope bias (rad/s)(VNED)
mag_bias = state(26:28);             % magnetometer bias (uT)(NED)

end

== matlab function car_model/Control Systems/Sensor Fusion/SNED to VNED ==
  data: accel_VNED output size=[3 1]; gyro_VNED output size=[3 1]; accel_SNED input; gyro_SNED input; mag_SNED input; mag_VNED output size=[3 1]; phi parameter
function [accel_VNED, gyro_VNED, mag_VNED] = SNED2VNED(accel_SNED, gyro_SNED, mag_SNED, phi)
%% Define Rotation
IMUNED2VNED = rotmat(quaternion([0 (phi - 180) 0],"eulerd","XYZ","frame"),"frame");
MAGNED2VNED = rotmat(quaternion([180 (180 - phi) 0],"eulerd","XYZ","frame"),"frame");

%% Coordinate Transformation
accel_VNED = IMUNED2VNED*accel_SNED;  % chassis acceleration (m/s^2)(NED)
gyro_VNED = IMUNED2VNED*gyro_SNED;    % chassis angular velocity (rad/s)(VNED)
mag_VNED = MAGNED2VNED*mag_SNED;      % magnetic field (uT)(NED)

end
